simulink model "sldemo_raccel_engine_idle_speed"  (Simulink 7.6)
settings: Solver=ode45  StartTime=0  StopTime=150  RelTol=1e-3
PreLoadFcn:
  | load sldemo_raccel_engine_idle_speed_data.mat
undefined symbols (not defined in the file or in its folder): damp1, damp2, damp3, delay, freq1, freq2, freq3, gain1, gain2, gain3, meanSpeed
settings Model: Creator=The MathWorks Inc.  SimulationMode=rapid-accelerator  ExtModeAutoUpdateStatusClock=off  TunableVars=gain2,gain3  TunableVarsStorageClass=Auto,Auto  TunableVarsTypeQualifier=,
settings DataIOCC: LimitDataPoints=off  SaveOutput=off  SaveTime=off  SignalLoggingName=logsOut
settings OptimizationCC: BooleanDataType=off  InlineParams=on  InlineInvariantSignals=on  InitFltsAndDblsToZero=on  EfficientMapNaN2IntZero=off
settings DebuggingCC: SaveWithParameterizedLinksMsg=none  CheckExecutionContextPreStartOutputMsg=on  CheckExecutionContextRuntimeOutputMsg=on  SignalResolutionControl=TryResolveAllWithWarning  SolverPrmCheckMsg=none  MultiTaskDSMMsg=warning  MultiTaskCondExecSysMsg=none
settings HardwareCC: TargetUnknown=on
settings ModelReferenceCC: UpdateModelReferenceTargets=IfOutOfDate
settings RTWCC: ProfileTLC=on  IncludeERTFirstTime=on
settings GRTTargetCC: TargetFcnLib=ansi_tfl_tmw.mat

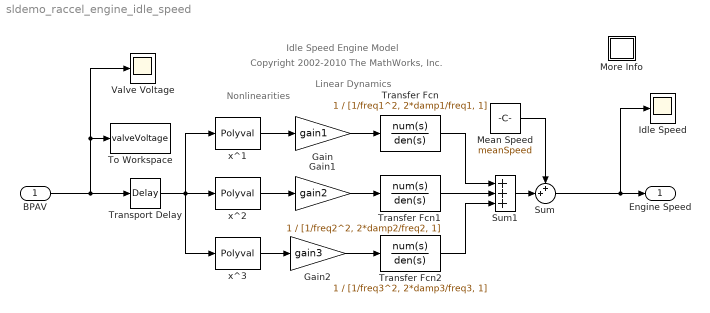
== system sldemo_raccel_engine_idle_speed ==
  note: Idle Speed Engine Model
  note: Nonlinearities
  note: Copyright 2002-2010 The MathWorks, Inc.
  note: Linear Dynamics
  BPAV : Inport
  Gain : Gain  Gain=gain1
  Gain1 : Gain  Gain=gain2
  Gain2 : Gain  Gain=gain3
  Idle Speed : Scope
      settings: TickLabels=on  TimeRange=150  YMin=600  YMax=950  DataFormat=Array
  Mean Speed : Constant  Value=meanSpeed
  More Info : Subsystem
      settings: OpenFcn=showdemo('sldemo_parallel_rapid_accel_sims_script')
      mask Display: disp('?')
  Sum : Sum  Inputs=++|
  Sum1 : Sum  Inputs=+++
  To Workspace : ToWorkspace  VariableName=valveVoltage  SampleTime=-1  SaveFormat=Array
  Transfer Fcn : TransferFcn  Numerator=1  Denominator=[1/freq1^2, 2*damp1/freq1, 1]
  Transfer Fcn1 : TransferFcn  Numerator=1  Denominator=[1/freq2^2, 2*damp2/freq2, 1]
  Transfer Fcn2 : TransferFcn  Numerator=1  Denominator=[1/freq3^2, 2*damp3/freq3, 1]
  Transport Delay : TransportDelay  DelayTime=delay  PadeOrder=1
  Valve Voltage : Scope
      settings: TickLabels=on  TimeRange=150  YMin=-1.5  YMax=1.5  DataFormat=Array
  x^1 : Polyval  Coefs=[1 0]
  x^2 : Polyval  Coefs=[1 0 0]
  x^3 : Polyval  Coefs=[1 0 0 0]
  Engine Speed : Outport
  wires:
  BPAV/1 -> Transport Delay/1, Valve Voltage/1, To Workspace/1
  Transfer Fcn/1 -> Sum1/1
  Transfer Fcn1/1 -> Sum1/2
  Transfer Fcn2/1 -> Sum1/3
  x^1/1 -> Gain/1
  x^3/1 -> Gain2/1
  x^2/1 -> Gain1/1
  Transport Delay/1 -> x^2/1, x^1/1, x^3/1
  Sum1/1 -> Sum/2
  Mean Speed/1 -> Sum/1
  Sum/1 -> Engine Speed/1, Idle Speed/1
  Gain/1 -> Transfer Fcn/1
  Gain1/1 -> Transfer Fcn1/1
  Gain2/1 -> Transfer Fcn2/1

== system sldemo_raccel_engine_idle_speed/More Info ==
